simulink model "structuri_avansate_de_control"  (R2022b)
settings: Solver=FixedStepAuto  StartTime=0.0  StopTime=900  FixedStep=0.01  RelTol=1e-3
values from neighbouring files (symbols this model uses):
  C = 5.6    [CalculeProiect.m]
  h0 = 13.97    [CalculeProiect.m]
  h1 = 17.85    [CalculeProiect.m]
  k = 0.024    [CalculeProiect.m]
  k1 = 0.624    [CalculeProiect.m]
  k11 = k2*k2+4*(k-k3)*k1    (= 0.0616266)    [CalculeProiect.m]
  k12 = 8*(k-k3)    (= 0.1968)    [CalculeProiect.m]
  k13 = 2*(k-k3)    (= 0.0492)    [CalculeProiect.m]
  k2 = -0.015    [CalculeProiect.m]
  k3 = -0.0006    [CalculeProiect.m]
  kcompensare = (delta_h/(q1-q0))/(delta_h/delta_ua)    (= 0.185185185185)    [CalculeProiect.m]
  kp = (delta_h/3)/delta_ua    (= 2.58666666667)    [CalculeProiect.m]
  q0 = 20.97    [CalculeProiect.m]
undefined symbols (not defined in the file or in its folder): ki, ki1, ki2, kp1, kp2
libraries: slpidlib x6
(part 1 of 2)
settings Model: Creator=denis  LastModifiedBy=denis

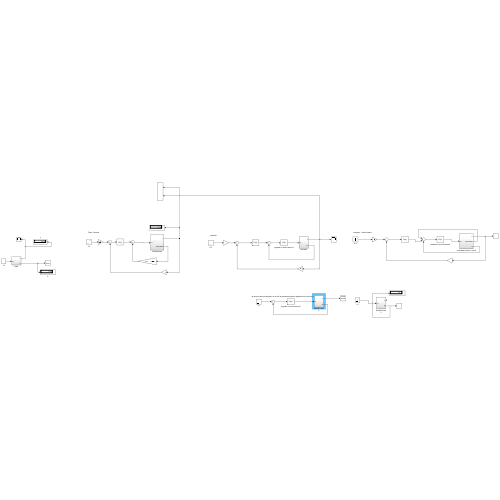
[thumbnail: Simulink's stored preview of the top-level diagram]
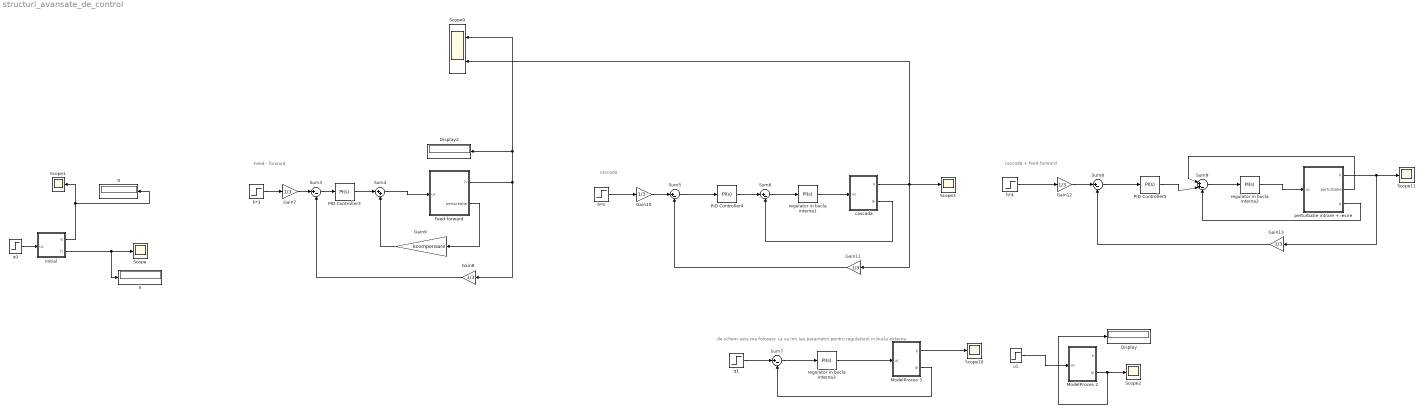
== system structuri_avansate_de_control ==
  note: de schem asta ma folosesc ca sa imi iau parametrii pentru regulatorul in bucla externa
  note: cascada
  note: Feed - forward
  note: cascada + feed-forward
  Display : Display
  Display2 : Display
  Feed-forward : Subsystem
  Gain{7..8,10..13} (6 alike) : Gain  Gain=1/3
  Gain9 : Gain  Gain=kcompensare
  ModelProces 2 : Subsystem
  ModelProces 3 : Subsystem
  PID Controller3 : slpidlib/PID Controller  Controller=PI  Form=Parallel  TimeDomain=Continuous-time  UseExternalTs=off  SampleTime=-1  IntegratorMethod=Forward Euler  FilterMethod=Forward Euler  ControllerParametersSource=internal  P=kp  I=ki  UseKiTs=off  D=0  N=100  UseFilter=on  TunerSelectOption=Transfer Function Based (PID Tuner App)  InitialConditionSource=internal  InitialConditionForIntegrator=4.4  InitialConditionForFilter=0  DifferentiatorICPrevScaledInput=0  ExternalReset=none  TrackingMode=off  Kt=1  LimitOutput=off  SatLimitsSource=internal  UpperSaturationLimit=inf  LowerSaturationLimit=-inf  LinearizeAsGain=on  AntiWindupMode=none  Kb=1  LimitIntegrator=off  UpperIntegratorSaturationLimit=inf  LowerIntegratorSaturationLimit=-inf  POutMin=[]  POutMax=[]  IOutMin=[]  IOutMax=[]  DOutMin=[]  DOutMax=[]  NOutMin=[]  NOutMax=[]  SumOutMin=[]  SumOutMax=[]  SaturationOutMin=[]  SaturationOutMax=[]  PParamMin=[]  PParamMax=[]  IParamMin=[]  IParamMax=[]  DParamMin=[]  DParamMax=[]  NParamMin=[]  NParamMax=[]  KbParamMin=[]  KbParamMax=[]  KtParamMin=[]  KtParamMax=[]  KbOutMin=[]  KbOutMax=[]  KtOutMin=[]  KtOutMax=[]  IntegratorOutMin=[]  IntegratorOutMax=[]  FilterOutMin=[]  FilterOutMax=[]  SumI1OutMin=[]  SumI1OutMax=[]  SumI2OutMin=[]  SumI2OutMax=[]  SumI3OutMin=[]  SumI3OutMax=[]  SumI4OutMin=[]  SumI4OutMax=[]  SumDOutMin=[]  SumDOutMax=[]  DifferentiatorOutMin=[]  DifferentiatorOutMax=[]  FilterDiffOutCoefMin=[]  FilterDiffOutCoefMax=[]  ReciprocalOutMin=[]  ReciprocalOutMax=[]  SumDenOutMin=[]  SumDenOutMax=[]  SumNumOutMin=[]  SumNumOutMax=[]  DivideOutMin=[]  DivideOutMax=[]  UdiffTsProdOutMin=[]  UdiffTsProdOutMax=[]  NTsProdOutMin=[]  NTsProdOutMax=[]  UintegralTsProdOutMin=[]  UintegralTsProdOutMax=[]  UngainTsProdOutMin=[]  UngainTsProdOutMax=[]  ClampingZeroOutDataTypeStr=Inherit: Inherit via back propagation  ClampingZeroOutMin=[]  ClampingZeroOutMax=[]  FilterDenConstantOutDataTypeStr=Inherit: Inherit via back propagation  FilterDenConstantOutMin=[]  FilterDenConstantOutMax=[]  PCopyOutDataTypeStr=Inherit: Inherit via back propagation  PCopyOutMin=[]  PCopyOutMax=[]  NCopyOutDataTypeStr=Inherit: Inherit via back propagation  NCopyOutMin=[]  NCopyOutMax=[]  IntegratorContinuousStateAttributes=''  IntegratorStateMustResolveToSignalObject=off  IntegratorRTWStateStorageClass=Auto  FilterContinuousStateAttributes=''  FilterStateMustResolveToSignalObject=off  FilterRTWStateStorageClass=Auto  ParallelPVariant=InternalParameters  IdealPVariant=Disabled  IVariant=InternalParameters  DVariant=Disabled  IntegratorVariant=Continuous  SatVariant=Disabled  AWVariant=Passthrough  PCopyVariant=Disabled  TRVariant=Disabled  FdbkBlocksVariant=Forward  IdealPFdbkVariant=Disabled  SatFdbkVariant=Disabled  DerivativeFilterVariant=Disabled  NVariant=Disabled  NCopyVariant=Disabled_SignalSpec  FilterICVariant=Disabled  IntegratorICVariant=InternalICs  ExternalResetVariant=Disabled  TRSumVariant=Passthrough  SumFdbkVariant=Disabled  SumVariant=Sum_PI  TsampFilterVariant=InternalTs  TsampNgainVariant=Passthrough  TsampIntegralVariant=Passthrough  ExternalSaturationOutDataTypeStr=Inherit: Same as second input
  PID Controller4 : slpidlib/PID Controller  Controller=PI  Form=Parallel  TimeDomain=Continuous-time  UseExternalTs=off  SampleTime=-1  IntegratorMethod=Forward Euler  FilterMethod=Forward Euler  ControllerParametersSource=internal  P=kp2  I=ki2  UseKiTs=off  D=0  N=100  UseFilter=on  TunerSelectOption=Transfer Function Based (PID Tuner App)  InitialConditionSource=internal  InitialConditionForIntegrator=20.97  InitialConditionForFilter=0  DifferentiatorICPrevScaledInput=0  ExternalReset=none  TrackingMode=off  Kt=1  LimitOutput=off  SatLimitsSource=internal  UpperSaturationLimit=inf  LowerSaturationLimit=-inf  LinearizeAsGain=on  AntiWindupMode=none  Kb=1  LimitIntegrator=off  UpperIntegratorSaturationLimit=inf  LowerIntegratorSaturationLimit=-inf  POutMin=[]  POutMax=[]  IOutMin=[]  IOutMax=[]  DOutMin=[]  DOutMax=[]  NOutMin=[]  NOutMax=[]  SumOutMin=[]  SumOutMax=[]  SaturationOutMin=[]  SaturationOutMax=[]  PParamMin=[]  PParamMax=[]  IParamMin=[]  IParamMax=[]  DParamMin=[]  DParamMax=[]  NParamMin=[]  NParamMax=[]  KbParamMin=[]  KbParamMax=[]  KtParamMin=[]  KtParamMax=[]  KbOutMin=[]  KbOutMax=[]  KtOutMin=[]  KtOutMax=[]  IntegratorOutMin=[]  IntegratorOutMax=[]  FilterOutMin=[]  FilterOutMax=[]  SumI1OutMin=[]  SumI1OutMax=[]  SumI2OutMin=[]  SumI2OutMax=[]  SumI3OutMin=[]  SumI3OutMax=[]  SumI4OutMin=[]  SumI4OutMax=[]  SumDOutMin=[]  SumDOutMax=[]  DifferentiatorOutMin=[]  DifferentiatorOutMax=[]  FilterDiffOutCoefMin=[]  FilterDiffOutCoefMax=[]  ReciprocalOutMin=[]  ReciprocalOutMax=[]  SumDenOutMin=[]  SumDenOutMax=[]  SumNumOutMin=[]  SumNumOutMax=[]  DivideOutMin=[]  DivideOutMax=[]  UdiffTsProdOutMin=[]  UdiffTsProdOutMax=[]  NTsProdOutMin=[]  NTsProdOutMax=[]  UintegralTsProdOutMin=[]  UintegralTsProdOutMax=[]  UngainTsProdOutMin=[]  UngainTsProdOutMax=[]  ClampingZeroOutDataTypeStr=Inherit: Inherit via back propagation  ClampingZeroOutMin=[]  ClampingZeroOutMax=[]  FilterDenConstantOutDataTypeStr=Inherit: Inherit via back propagation  FilterDenConstantOutMin=[]  FilterDenConstantOutMax=[]  PCopyOutDataTypeStr=Inherit: Inherit via back propagation  PCopyOutMin=[]  PCopyOutMax=[]  NCopyOutDataTypeStr=Inherit: Inherit via back propagation  NCopyOutMin=[]  NCopyOutMax=[]  IntegratorContinuousStateAttributes=''  IntegratorStateMustResolveToSignalObject=off  IntegratorRTWStateStorageClass=Auto  FilterContinuousStateAttributes=''  FilterStateMustResolveToSignalObject=off  FilterRTWStateStorageClass=Auto  ParallelPVariant=InternalParameters  IdealPVariant=Disabled  IVariant=InternalParameters  DVariant=Disabled  IntegratorVariant=Continuous  SatVariant=Disabled  AWVariant=Passthrough  PCopyVariant=Disabled  TRVariant=Disabled  FdbkBlocksVariant=Forward  IdealPFdbkVariant=Disabled  SatFdbkVariant=Disabled  DerivativeFilterVariant=Disabled  NVariant=Disabled  NCopyVariant=Disabled_SignalSpec  FilterICVariant=Disabled  IntegratorICVariant=InternalICs  ExternalResetVariant=Disabled  TRSumVariant=Passthrough  SumFdbkVariant=Disabled  SumVariant=Sum_PI  TsampFilterVariant=InternalTs  TsampNgainVariant=Passthrough  TsampIntegralVariant=Passthrough  ExternalSaturationOutDataTypeStr=Inherit: Same as second input
  PID Controller5 : slpidlib/PID Controller  Controller=PI  Form=Parallel  TimeDomain=Continuous-time  UseExternalTs=off  SampleTime=-1  IntegratorMethod=Forward Euler  FilterMethod=Forward Euler  ControllerParametersSource=internal  P=kp2  I=ki2  UseKiTs=off  D=0  N=100  UseFilter=on  TunerSelectOption=Transfer Function Based (PID Tuner App)  InitialConditionSource=internal  InitialConditionForIntegrator=q0  InitialConditionForFilter=0  DifferentiatorICPrevScaledInput=0  ExternalReset=none  TrackingMode=off  Kt=1  LimitOutput=off  SatLimitsSource=internal  UpperSaturationLimit=inf  LowerSaturationLimit=-inf  LinearizeAsGain=on  AntiWindupMode=none  Kb=1  LimitIntegrator=off  UpperIntegratorSaturationLimit=inf  LowerIntegratorSaturationLimit=-inf  POutMin=[]  POutMax=[]  IOutMin=[]  IOutMax=[]  DOutMin=[]  DOutMax=[]  NOutMin=[]  NOutMax=[]  SumOutMin=[]  SumOutMax=[]  SaturationOutMin=[]  SaturationOutMax=[]  PParamMin=[]  PParamMax=[]  IParamMin=[]  IParamMax=[]  DParamMin=[]  DParamMax=[]  NParamMin=[]  NParamMax=[]  KbParamMin=[]  KbParamMax=[]  KtParamMin=[]  KtParamMax=[]  KbOutMin=[]  KbOutMax=[]  KtOutMin=[]  KtOutMax=[]  IntegratorOutMin=[]  IntegratorOutMax=[]  FilterOutMin=[]  FilterOutMax=[]  SumI1OutMin=[]  SumI1OutMax=[]  SumI2OutMin=[]  SumI2OutMax=[]  SumI3OutMin=[]  SumI3OutMax=[]  SumI4OutMin=[]  SumI4OutMax=[]  SumDOutMin=[]  SumDOutMax=[]  DifferentiatorOutMin=[]  DifferentiatorOutMax=[]  FilterDiffOutCoefMin=[]  FilterDiffOutCoefMax=[]  ReciprocalOutMin=[]  ReciprocalOutMax=[]  SumDenOutMin=[]  SumDenOutMax=[]  SumNumOutMin=[]  SumNumOutMax=[]  DivideOutMin=[]  DivideOutMax=[]  UdiffTsProdOutMin=[]  UdiffTsProdOutMax=[]  NTsProdOutMin=[]  NTsProdOutMax=[]  UintegralTsProdOutMin=[]  UintegralTsProdOutMax=[]  UngainTsProdOutMin=[]  UngainTsProdOutMax=[]  ClampingZeroOutDataTypeStr=Inherit: Inherit via back propagation  ClampingZeroOutMin=[]  ClampingZeroOutMax=[]  FilterDenConstantOutDataTypeStr=Inherit: Inherit via back propagation  FilterDenConstantOutMin=[]  FilterDenConstantOutMax=[]  PCopyOutDataTypeStr=Inherit: Inherit via back propagation  PCopyOutMin=[]  PCopyOutMax=[]  NCopyOutDataTypeStr=Inherit: Inherit via back propagation  NCopyOutMin=[]  NCopyOutMax=[]  IntegratorContinuousStateAttributes=''  IntegratorStateMustResolveToSignalObject=off  IntegratorRTWStateStorageClass=Auto  FilterContinuousStateAttributes=''  FilterStateMustResolveToSignalObject=off  FilterRTWStateStorageClass=Auto  ParallelPVariant=InternalParameters  IdealPVariant=Disabled  IVariant=InternalParameters  DVariant=Disabled  IntegratorVariant=Continuous  SatVariant=Disabled  AWVariant=Passthrough  PCopyVariant=Disabled  TRVariant=Disabled  FdbkBlocksVariant=Forward  IdealPFdbkVariant=Disabled  SatFdbkVariant=Disabled  DerivativeFilterVariant=Disabled  NVariant=Disabled  NCopyVariant=Disabled_SignalSpec  FilterICVariant=Disabled  IntegratorICVariant=InternalICs  ExternalResetVariant=Disabled  TRSumVariant=Passthrough  SumFdbkVariant=Disabled  SumVariant=Sum_PI  TsampFilterVariant=InternalTs  TsampNgainVariant=Passthrough  TsampIntegralVariant=Passthrough  ExternalSaturationOutDataTypeStr=Inherit: Same as second input
  Scope{,1..3,10..11} (6 alike) : Scope
  Scope9 : Scope  NumInputPorts=2
  Sum{3,5..8} (5 alike) : Sum  Inputs=|+-
  Sum4 : Sum  Inputs=|++
  Sum9 : Sum  Inputs=|++-
  cascada : Subsystem
  h : Display
  h*3 : Step  Before=h0  After=h1  SampleTime=0
  h*4 : Step  Time=0  Before=h0  After=h1  SampleTime=0
  h*5 : Step  Time=0  Before=h0  After=h1  SampleTime=0
  initial : Subsystem
  perturbatie intrare + iesire : Subsystem
  q : Display
  q1 : Step  Time=0  Before=q0  After=29.02  SampleTime=0
  regulator in bucla interna1 : slpidlib/PID Controller  Controller=PI  Form=Parallel  TimeDomain=Continuous-time  UseExternalTs=off  SampleTime=-1  IntegratorMethod=Forward Euler  FilterMethod=Forward Euler  ControllerParametersSource=internal  P=kp1  I=ki1  UseKiTs=off  D=0  N=100  UseFilter=on  TunerSelectOption=Transfer Function Based (PID Tuner App)  InitialConditionSource=internal  InitialConditionForIntegrator=4.4  InitialConditionForFilter=0  DifferentiatorICPrevScaledInput=0  ExternalReset=none  TrackingMode=off  Kt=1  LimitOutput=off  SatLimitsSource=internal  UpperSaturationLimit=inf  LowerSaturationLimit=-inf  LinearizeAsGain=on  AntiWindupMode=none  Kb=1  LimitIntegrator=off  UpperIntegratorSaturationLimit=inf  LowerIntegratorSaturationLimit=-inf  POutMin=[]  POutMax=[]  IOutMin=[]  IOutMax=[]  DOutMin=[]  DOutMax=[]  NOutMin=[]  NOutMax=[]  SumOutMin=[]  SumOutMax=[]  SaturationOutMin=[]  SaturationOutMax=[]  PParamMin=[]  PParamMax=[]  IParamMin=[]  IParamMax=[]  DParamMin=[]  DParamMax=[]  NParamMin=[]  NParamMax=[]  KbParamMin=[]  KbParamMax=[]  KtParamMin=[]  KtParamMax=[]  KbOutMin=[]  KbOutMax=[]  KtOutMin=[]  KtOutMax=[]  IntegratorOutMin=[]  IntegratorOutMax=[]  FilterOutMin=[]  FilterOutMax=[]  SumI1OutMin=[]  SumI1OutMax=[]  SumI2OutMin=[]  SumI2OutMax=[]  SumI3OutMin=[]  SumI3OutMax=[]  SumI4OutMin=[]  SumI4OutMax=[]  SumDOutMin=[]  SumDOutMax=[]  DifferentiatorOutMin=[]  DifferentiatorOutMax=[]  FilterDiffOutCoefMin=[]  FilterDiffOutCoefMax=[]  ReciprocalOutMin=[]  ReciprocalOutMax=[]  SumDenOutMin=[]  SumDenOutMax=[]  SumNumOutMin=[]  SumNumOutMax=[]  DivideOutMin=[]  DivideOutMax=[]  UdiffTsProdOutMin=[]  UdiffTsProdOutMax=[]  NTsProdOutMin=[]  NTsProdOutMax=[]  UintegralTsProdOutMin=[]  UintegralTsProdOutMax=[]  UngainTsProdOutMin=[]  UngainTsProdOutMax=[]  ClampingZeroOutDataTypeStr=Inherit: Inherit via back propagation  ClampingZeroOutMin=[]  ClampingZeroOutMax=[]  FilterDenConstantOutDataTypeStr=Inherit: Inherit via back propagation  FilterDenConstantOutMin=[]  FilterDenConstantOutMax=[]  PCopyOutDataTypeStr=Inherit: Inherit via back propagation  PCopyOutMin=[]  PCopyOutMax=[]  NCopyOutDataTypeStr=Inherit: Inherit via back propagation  NCopyOutMin=[]  NCopyOutMax=[]  IntegratorContinuousStateAttributes=''  IntegratorStateMustResolveToSignalObject=off  IntegratorRTWStateStorageClass=Auto  FilterContinuousStateAttributes=''  FilterStateMustResolveToSignalObject=off  FilterRTWStateStorageClass=Auto  ParallelPVariant=InternalParameters  IdealPVariant=Disabled  IVariant=InternalParameters  DVariant=Disabled  IntegratorVariant=Continuous  SatVariant=Disabled  AWVariant=Passthrough  PCopyVariant=Disabled  TRVariant=Disabled  FdbkBlocksVariant=Forward  IdealPFdbkVariant=Disabled  SatFdbkVariant=Disabled  DerivativeFilterVariant=Disabled  NVariant=Disabled  NCopyVariant=Disabled_SignalSpec  FilterICVariant=Disabled  IntegratorICVariant=InternalICs  ExternalResetVariant=Disabled  TRSumVariant=Passthrough  SumFdbkVariant=Disabled  SumVariant=Sum_PI  TsampFilterVariant=InternalTs  TsampNgainVariant=Passthrough  TsampIntegralVariant=Passthrough  ExternalSaturationOutDataTypeStr=Inherit: Same as second input
  regulator in bucla interna2 : slpidlib/PID Controller  Controller=PI  Form=Parallel  TimeDomain=Continuous-time  UseExternalTs=off  SampleTime=-1  IntegratorMethod=Forward Euler  FilterMethod=Forward Euler  ControllerParametersSource=internal  P=kp1  I=ki1  UseKiTs=off  D=0  N=100  UseFilter=on  TunerSelectOption=Transfer Function Based (PID Tuner App)  InitialConditionSource=internal  InitialConditionForIntegrator=4.4  InitialConditionForFilter=0  DifferentiatorICPrevScaledInput=0  ExternalReset=none  TrackingMode=off  Kt=1  LimitOutput=off  SatLimitsSource=internal  UpperSaturationLimit=inf  LowerSaturationLimit=-inf  LinearizeAsGain=on  AntiWindupMode=none  Kb=1  LimitIntegrator=off  UpperIntegratorSaturationLimit=inf  LowerIntegratorSaturationLimit=-inf  POutMin=[]  POutMax=[]  IOutMin=[]  IOutMax=[]  DOutMin=[]  DOutMax=[]  NOutMin=[]  NOutMax=[]  SumOutMin=[]  SumOutMax=[]  SaturationOutMin=[]  SaturationOutMax=[]  PParamMin=[]  PParamMax=[]  IParamMin=[]  IParamMax=[]  DParamMin=[]  DParamMax=[]  NParamMin=[]  NParamMax=[]  KbParamMin=[]  KbParamMax=[]  KtParamMin=[]  KtParamMax=[]  KbOutMin=[]  KbOutMax=[]  KtOutMin=[]  KtOutMax=[]  IntegratorOutMin=[]  IntegratorOutMax=[]  FilterOutMin=[]  FilterOutMax=[]  SumI1OutMin=[]  SumI1OutMax=[]  SumI2OutMin=[]  SumI2OutMax=[]  SumI3OutMin=[]  SumI3OutMax=[]  SumI4OutMin=[]  SumI4OutMax=[]  SumDOutMin=[]  SumDOutMax=[]  DifferentiatorOutMin=[]  DifferentiatorOutMax=[]  FilterDiffOutCoefMin=[]  FilterDiffOutCoefMax=[]  ReciprocalOutMin=[]  ReciprocalOutMax=[]  SumDenOutMin=[]  SumDenOutMax=[]  SumNumOutMin=[]  SumNumOutMax=[]  DivideOutMin=[]  DivideOutMax=[]  UdiffTsProdOutMin=[]  UdiffTsProdOutMax=[]  NTsProdOutMin=[]  NTsProdOutMax=[]  UintegralTsProdOutMin=[]  UintegralTsProdOutMax=[]  UngainTsProdOutMin=[]  UngainTsProdOutMax=[]  ClampingZeroOutDataTypeStr=Inherit: Inherit via back propagation  ClampingZeroOutMin=[]  ClampingZeroOutMax=[]  FilterDenConstantOutDataTypeStr=Inherit: Inherit via back propagation  FilterDenConstantOutMin=[]  FilterDenConstantOutMax=[]  PCopyOutDataTypeStr=Inherit: Inherit via back propagation  PCopyOutMin=[]  PCopyOutMax=[]  NCopyOutDataTypeStr=Inherit: Inherit via back propagation  NCopyOutMin=[]  NCopyOutMax=[]  IntegratorContinuousStateAttributes=''  IntegratorStateMustResolveToSignalObject=off  IntegratorRTWStateStorageClass=Auto  FilterContinuousStateAttributes=''  FilterStateMustResolveToSignalObject=off  FilterRTWStateStorageClass=Auto  ParallelPVariant=InternalParameters  IdealPVariant=Disabled  IVariant=InternalParameters  DVariant=Disabled  IntegratorVariant=Continuous  SatVariant=Disabled  AWVariant=Passthrough  PCopyVariant=Disabled  TRVariant=Disabled  FdbkBlocksVariant=Forward  IdealPFdbkVariant=Disabled  SatFdbkVariant=Disabled  DerivativeFilterVariant=Disabled  NVariant=Disabled  NCopyVariant=Disabled_SignalSpec  FilterICVariant=Disabled  IntegratorICVariant=InternalICs  ExternalResetVariant=Disabled  TRSumVariant=Passthrough  SumFdbkVariant=Disabled  SumVariant=Sum_PI  TsampFilterVariant=InternalTs  TsampNgainVariant=Passthrough  TsampIntegralVariant=Passthrough  ExternalSaturationOutDataTypeStr=Inherit: Same as second input
  regulator in bucla interna3 : slpidlib/PID Controller  Controller=PI  Form=Parallel  TimeDomain=Continuous-time  UseExternalTs=off  SampleTime=-1  IntegratorMethod=Forward Euler  FilterMethod=Forward Euler  ControllerParametersSource=internal  P=kp1  I=ki1  UseKiTs=off  D=0  N=100  UseFilter=on  TunerSelectOption=Transfer Function Based (PID Tuner App)  InitialConditionSource=internal  InitialConditionForIntegrator=4.4  InitialConditionForFilter=0  DifferentiatorICPrevScaledInput=0  ExternalReset=none  TrackingMode=off  Kt=1  LimitOutput=off  SatLimitsSource=internal  UpperSaturationLimit=inf  LowerSaturationLimit=-inf  LinearizeAsGain=on  AntiWindupMode=none  Kb=1  LimitIntegrator=off  UpperIntegratorSaturationLimit=inf  LowerIntegratorSaturationLimit=-inf  POutMin=[]  POutMax=[]  IOutMin=[]  IOutMax=[]  DOutMin=[]  DOutMax=[]  NOutMin=[]  NOutMax=[]  SumOutMin=[]  SumOutMax=[]  SaturationOutMin=[]  SaturationOutMax=[]  PParamMin=[]  PParamMax=[]  IParamMin=[]  IParamMax=[]  DParamMin=[]  DParamMax=[]  NParamMin=[]  NParamMax=[]  KbParamMin=[]  KbParamMax=[]  KtParamMin=[]  KtParamMax=[]  KbOutMin=[]  KbOutMax=[]  KtOutMin=[]  KtOutMax=[]  IntegratorOutMin=[]  IntegratorOutMax=[]  FilterOutMin=[]  FilterOutMax=[]  SumI1OutMin=[]  SumI1OutMax=[]  SumI2OutMin=[]  SumI2OutMax=[]  SumI3OutMin=[]  SumI3OutMax=[]  SumI4OutMin=[]  SumI4OutMax=[]  SumDOutMin=[]  SumDOutMax=[]  DifferentiatorOutMin=[]  DifferentiatorOutMax=[]  FilterDiffOutCoefMin=[]  FilterDiffOutCoefMax=[]  ReciprocalOutMin=[]  ReciprocalOutMax=[]  SumDenOutMin=[]  SumDenOutMax=[]  SumNumOutMin=[]  SumNumOutMax=[]  DivideOutMin=[]  DivideOutMax=[]  UdiffTsProdOutMin=[]  UdiffTsProdOutMax=[]  NTsProdOutMin=[]  NTsProdOutMax=[]  UintegralTsProdOutMin=[]  UintegralTsProdOutMax=[]  UngainTsProdOutMin=[]  UngainTsProdOutMax=[]  ClampingZeroOutDataTypeStr=Inherit: Inherit via back propagation  ClampingZeroOutMin=[]  ClampingZeroOutMax=[]  FilterDenConstantOutDataTypeStr=Inherit: Inherit via back propagation  FilterDenConstantOutMin=[]  FilterDenConstantOutMax=[]  PCopyOutDataTypeStr=Inherit: Inherit via back propagation  PCopyOutMin=[]  PCopyOutMax=[]  NCopyOutDataTypeStr=Inherit: Inherit via back propagation  NCopyOutMin=[]  NCopyOutMax=[]  IntegratorContinuousStateAttributes=''  IntegratorStateMustResolveToSignalObject=off  IntegratorRTWStateStorageClass=Auto  FilterContinuousStateAttributes=''  FilterStateMustResolveToSignalObject=off  FilterRTWStateStorageClass=Auto  ParallelPVariant=InternalParameters  IdealPVariant=Disabled  IVariant=InternalParameters  DVariant=Disabled  IntegratorVariant=Continuous  SatVariant=Disabled  AWVariant=Passthrough  PCopyVariant=Disabled  TRVariant=Disabled  FdbkBlocksVariant=Forward  IdealPFdbkVariant=Disabled  SatFdbkVariant=Disabled  DerivativeFilterVariant=Disabled  NVariant=Disabled  NCopyVariant=Disabled_SignalSpec  FilterICVariant=Disabled  IntegratorICVariant=InternalICs  ExternalResetVariant=Disabled  TRSumVariant=Passthrough  SumFdbkVariant=Disabled  SumVariant=Sum_PI  TsampFilterVariant=InternalTs  TsampNgainVariant=Passthrough  TsampIntegralVariant=Passthrough  ExternalSaturationOutDataTypeStr=Inherit: Same as second input
  u0 : Step  Time=0  Before=4.4  After=4.9  SampleTime=0
  u1 : Step  Time=0  Before=4.4  After=4.9  SampleTime=0
  wires:
  Sum4/1 -> Feed-forward/1(uc)
  ModelProces 3/2(qi) -> Sum7/2
  cascada/1(h) -> Scope9/2, Scope3/1, Gain11/1
  ModelProces 2/2(qi) -> Display/1, Scope2/1
  Sum3/1 -> PID Controller3/1
  Gain12/1 -> Sum8/1
  Sum9/1 -> regulator in bucla interna2/1
  Gain11/1 -> Sum5/2
  regulator in bucla interna3/1 -> ModelProces 3/1(uc)
  initial/2(h) -> Scope/1, h/1
  Feed-forward/2(perturbatie) -> Gain9/1
  PID Controller3/1 -> Sum4/1
  Gain10/1 -> Sum5/1
  initial/1(q) -> Scope1/1, q/1
  h*3/1 -> Gain7/1
  Gain7/1 -> Sum3/1
  Sum6/1 -> regulator in bucla interna1/1
  regulator in bucla interna1/1 -> cascada/1(uc)
  ModelProces 3/1(h) -> Scope10/1
  perturbatie intrare + iesire/1(h) -> Gain13/1, Scope11/1
  h*5/1 -> Gain10/1
  Sum5/1 -> PID Controller4/1
  q1/1 -> Sum7/1
  Gain13/1 -> Sum8/2
  Gain8/1 -> Sum3/2
  PID Controller4/1 -> Sum6/1
  Sum7/1 -> regulator in bucla interna3/1
  perturbatie intrare + iesire/3(q) -> Sum9/3
  u1/1 -> ModelProces 2/1(uc)
  perturbatie intrare + iesire/2(perturbatie) -> Sum9/1
  u0/1 -> initial/1(uc)
  Gain9/1 -> Sum4/2
  Sum8/1 -> PID Controller5/1
  cascada/2(qi) -> Sum6/2
  Feed-forward/1(h) -> Gain8/1, Scope9/1, Display2/1
  regulator in bucla interna2/1 -> perturbatie intrare + iesire/1(uc)
  PID Controller5/1 -> Sum9/2
  h*4/1 -> Gain12/1

== system structuri_avansate_de_control/Feed-forward ==
  uc : Inport
  Amplificator : Subsystem
  Curent rotoric : Subsystem
  Filtru : Subsystem
  Motor : Subsystem
  Pompa : Subsystem
  Randament pompa : Subsystem
  Rezervor : Subsystem
  h : Outport
  perturbatie : Outport  Port=2
  wires:
  Filtru/1(q2) -> Curent rotoric/2(q), Randament pompa/1(q), Rezervor/1(q)
  Rezervor/1(h) -> h/1, Curent rotoric/1(h), Pompa/2(h)
  Motor/1(kn) -> Pompa/1(kn)
  Curent rotoric/1(im) -> Motor/2(im)
  Amplificator/1(um) -> Motor/1(um), Curent rotoric/4(um), Randament pompa/2(um)
  uc/1 -> Amplificator/1(ua)
  Randament pompa/1(eta) -> Curent rotoric/3(eta)
  Pompa/1(q) -> Filtru/1(q1)
  Rezervor/2(perturbatie) -> perturbatie/1

== system structuri_avansate_de_control/ModelProces 2 ==
  uc : Inport
  "Amplificator " : Subsystem
  Curentul_rotoric : Subsystem
  Filtru : Subsystem
  "Motor " : Subsystem
  Pompa : Subsystem
  Randament : Subsystem
  Rezervor : Subsystem
  perturbatie k : Step  Time=300  After=0.03  SampleTime=0
  h : Outport
  qi : Outport  Port=2
  wires:
  "Amplificator "/1("um ") -> "Motor "/1(um), Randament/2(um), Curentul_rotoric/4(um)
  Filtru/1(q_f) -> Rezervor/1(q), qi/1, Randament/1("q "), Curentul_rotoric/1(q)
  Rezervor/1(h) -> h/1, Curentul_rotoric/3(h), Pompa/1(h)
  Curentul_rotoric/1(im) -> "Motor "/2(im)
  Randament/1("eta ") -> Curentul_rotoric/2(eta)
  uc/1 -> "Amplificator "/1(ua)
  Pompa/1(q) -> Filtru/1(q)
  perturbatie k/1 -> Pompa/2(perturbatie k)
  "Motor "/1(kn) -> Pompa/3(kn)

== system structuri_avansate_de_control/ModelProces 3 ==
  uc : Inport
  "Amplificator " : Subsystem
  Curentul_rotoric : Subsystem
  Filtru : Subsystem
  "Motor " : Subsystem
  Pompa : Subsystem
  Randament : Subsystem
  Rezervor : Subsystem
  perturbatie k : Step  Time=300  After=0.03  SampleTime=0
  h : Outport
  qi : Outport  Port=2
  wires:
  "Amplificator "/1("um ") -> "Motor "/1(um), Randament/2(um), Curentul_rotoric/4(um)
  Filtru/1(q_f) -> Rezervor/1(q), qi/1, Randament/1("q "), Curentul_rotoric/1(q)
  Rezervor/1(h) -> h/1, Curentul_rotoric/3(h), Pompa/1(h)
  Curentul_rotoric/1(im) -> "Motor "/2(im)
  Randament/1("eta ") -> Curentul_rotoric/2(eta)
  uc/1 -> "Amplificator "/1(ua)
  Pompa/1(q) -> Filtru/1(q)
  perturbatie k/1 -> Pompa/2(perturbatie k)
  "Motor "/1(kn) -> Pompa/3(kn)

== system structuri_avansate_de_control/cascada ==
  uc : Inport
  "Amplificator " : Subsystem
  Curentul_rotoric : Subsystem
  Filtru : Subsystem
  "Motor " : Subsystem
  Pompa : Subsystem
  Randament : Subsystem
  Rezervor : Subsystem
  perturbatie k : Step  Time=300  After=-0.02  SampleTime=0
  h : Outport
  qi : Outport  Port=2
  wires:
  "Amplificator "/1("um ") -> "Motor "/1(um), Randament/2(um), Curentul_rotoric/4(um)
  Filtru/1(q_f) -> Rezervor/1(q), qi/1, Randament/1("q "), Curentul_rotoric/1(q)
  Rezervor/1(h) -> h/1, Curentul_rotoric/3(h), Pompa/1(h)
  Curentul_rotoric/1(im) -> "Motor "/2(im)
  Randament/1("eta ") -> Curentul_rotoric/2(eta)
  uc/1 -> "Amplificator "/1(ua)
  Pompa/1(q) -> Filtru/1(q)
  perturbatie k/1 -> Pompa/2(perturbatie k)
  "Motor "/1(kn) -> Pompa/3(kn)

== system structuri_avansate_de_control/initial ==
  uc : Inport
  Amplificator : Subsystem
  Curent rotoric : Subsystem
  Filtru : Subsystem
  Motor : Subsystem
  Pompa : Subsystem
  Randament pompa : Subsystem
  Rezervor : Subsystem
  q : Outport
  h : Outport  Port=2
  wires:
  Filtru/1(q2) -> Curent rotoric/2(q), Randament pompa/1(q), Rezervor/1(ln1), q/1
  Rezervor/1(h) -> h/1, Curent rotoric/1(h), Pompa/2(h)
  Motor/1(kn) -> Pompa/1(kn)
  Curent rotoric/1(im) -> Motor/2(im)
  Amplificator/1(um) -> Motor/1(um), Curent rotoric/4(um), Randament pompa/2(um)
  uc/1 -> Amplificator/1(ua)
  Randament pompa/1(eta) -> Curent rotoric/3(eta)
  Pompa/1(q) -> Filtru/1(q1)

== system structuri_avansate_de_control/perturbatie intrare + iesire ==
  uc : Inport
  Amplificator : Subsystem
  Curent rotoric : Subsystem
  Filtru : Subsystem
  Motor : Subsystem
  Pompa : Subsystem
  Randament pompa : Subsystem
  Rezervor : Subsystem
  Step : Step  Time=300  After=-0.01  SampleTime=0
  h : Outport
  perturbatie : Outport  Port=2
  q : Outport  Port=3
  wires:
  Filtru/1(q2) -> Curent rotoric/2(q), Randament pompa/1(q), Rezervor/1(q), q/1
  Rezervor/1(h) -> h/1, Pompa/3(h), Curent rotoric/1(h)
  Curent rotoric/1(im) -> Motor/2(im)
  Amplificator/1(um) -> Motor/1(um), Curent rotoric/4(um), Randament pompa/2(um)
  uc/1 -> Amplificator/1(ua)
  Randament pompa/1(eta) -> Curent rotoric/3(eta)
  Pompa/1(q) -> Filtru/1(q1)
  Rezervor/2(perturbatie) -> perturbatie/1
  Motor/1(kn) -> Pompa/1(kn)
  Step/1 -> Pompa/2(perturbatie k)

== system structuri_avansate_de_control/Feed-forward/Amplificator ==
  ua : Inport
  Constant : Constant  Value=8.1
  Gain : Gain  Gain=2.2
  Gain1 : Gain  Gain=5
  Gain2 : Gain  Gain=2.2
  Saturation : Saturate  UpperLimit=22  LowerLimit=0
  Sum : Sum  Inputs=|++
  Sum1 : Sum  Inputs=|+-
  Switch : Switch  Criteria=u2 > Threshold  Threshold=8.1  SaturateOnIntegerOverflow=off  InputSameDT=off
  um : Outport
  wires:
  Gain/1 -> Switch/3
  Sum1/1 -> Gain1/1
  ua/1 -> Gain/1, Sum1/1, Gain2/1, Switch/2
  Switch/1 -> Saturation/1
  Gain1/1 -> Sum/2
  Saturation/1 -> um/1
  Constant/1 -> Sum1/2
  Gain2/1 -> Sum/1
  Sum/1 -> Switch/1

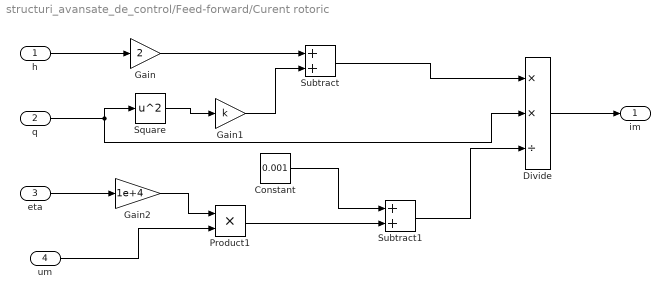
== system structuri_avansate_de_control/Feed-forward/Curent rotoric ==
  h : Inport
  q : Inport  Port=2
  eta : Inport  Port=3
  um : Inport  Port=4
  Constant : Constant  Value=0.001
  Divide : Product  Inputs=**/
  Gain : Gain  Gain=2
  Gain1 : Gain  Gain=k
  Gain2 : Gain  Gain=1e+4
  Product1 : Product
  Square : Math  Operator=square
  Subtract : Sum
  Subtract1 : Sum
  im : Outport
  wires:
  h/1 -> Gain/1
  Divide/1 -> im/1
  q/1 -> Divide/2, Square/1
  eta/1 -> Gain2/1
  um/1 -> Product1/2
  Gain2/1 -> Product1/1
  Subtract/1 -> Divide/1
  Constant/1 -> Subtract1/1
  Product1/1 -> Subtract1/2
  Subtract1/1 -> Divide/3
  Gain/1 -> Subtract/1
  Gain1/1 -> Subtract/2
  Square/1 -> Gain1/1

== system structuri_avansate_de_control/Feed-forward/Filtru ==
  q1 : Inport
  Integrator1 : Integrator  InitialCondition=q0
  Sum1 : Sum  Inputs=|+-
  q2 : Outport
  wires:
  Integrator1/1 -> q2/1, Sum1/2
  q1/1 -> Sum1/1
  Sum1/1 -> Integrator1/1

== system structuri_avansate_de_control/Feed-forward/Motor ==
  um : Inport
  im : Inport  Port=2
  Add : Sum  Inputs=+-
  Rm : Gain  Gain=3
  kn : Outport
  wires:
  Rm/1 -> Add/2
  um/1 -> Add/1
  im/1 -> Rm/1
  Add/1 -> kn/1

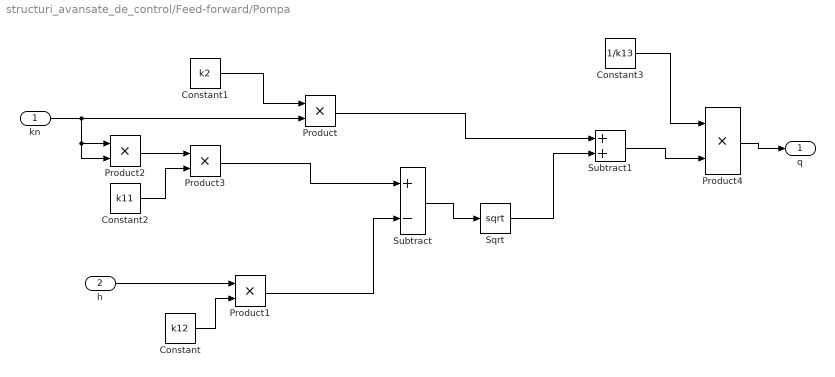
== system structuri_avansate_de_control/Feed-forward/Pompa ==
  kn : Inport
  h : Inport  Port=2
  Constant : Constant  Value=k12
  Constant1 : Constant  Value=k2
  Constant2 : Constant  Value=k11
  Constant3 : Constant  Value=1/k13
  Product{,1..4} (5 alike) : Product
  Sqrt : Sqrt
  Subtract : Sum  Inputs=+-
  Subtract1 : Sum
  q : Outport
  wires:
  Subtract/1 -> Sqrt/1
  Sqrt/1 -> Subtract1/2
  h/1 -> Product1/1
  Product1/1 -> Subtract/2
  Constant/1 -> Product1/2
  Constant1/1 -> Product/1
  kn/1 -> Product2/2, Product2/1, Product/2
  Product/1 -> Subtract1/1
  Product2/1 -> Product3/1
  Constant2/1 -> Product3/2
  Product3/1 -> Subtract/1
  Constant3/1 -> Product4/1
  Subtract1/1 -> Product4/2
  Product4/1 -> q/1

== system structuri_avansate_de_control/Feed-forward/Randament pompa ==
  q : Inport
  um : Inport  Port=2
  Gain : Gain  Gain=8e-5
  Product : Product
  eta : Outport
  wires:
  um/1 -> Gain/1
  Gain/1 -> Product/2
  q/1 -> Product/1
  Product/1 -> eta/1

== system structuri_avansate_de_control/Feed-forward/Rezervor ==
  q : Inport
  Add : Sum
  Constant : Constant  Value=C
  Gain : Gain  Gain=1/332.5
  Integrator1 : Integrator  InitialCondition=h0
  Product : Product
  Product1 : Product
  Scope : Scope
  Sqrt : Sqrt
  Step : Step  Time=500  After=0.11  SampleTime=0
  Sum1 : Sum  Inputs=|+-
  h : Outport
  perturbatie : Outport  Port=2
  wires:
  Gain/1 -> Integrator1/1
  Integrator1/1 -> Sqrt/1, h/1
  Sum1/1 -> Gain/1
  q/1 -> Sum1/1
  Sqrt/1 -> Product1/1, Product/1
  Product/1 -> Sum1/2, Scope/1
  Product1/1 -> perturbatie/1
  Constant/1 -> Add/2
  Step/1 -> Product1/2, Add/1
  Add/1 -> Product/2

== system structuri_avansate_de_control/ModelProces 2/Amplificator  ==
  ua : Inport
  Constant : Constant  Value=8.1
  Gain : Gain  Gain=2.2
  Gain1 : Gain  Gain=2.2
  Gain2 : Gain  Gain=5
  Saturation : Saturate  UpperLimit=22  LowerLimit=0
  Sum : Sum  Inputs=|++
  Sum1 : Sum  Inputs=|+-
  Switch : Switch  Threshold=8.1  SaturateOnIntegerOverflow=off  InputSameDT=off
  "um " : Outport
  wires:
  Sum1/1 -> Gain2/1
  ua/1 -> Switch/2, Gain/1, Sum1/1, Gain1/1
  Gain2/1 -> Sum/2
  Gain1/1 -> Sum/1
  Sum/1 -> Switch/1
  Gain/1 -> Switch/3
  Constant/1 -> Sum1/2
  Switch/1 -> Saturation/1
  Saturation/1 -> "um "/1

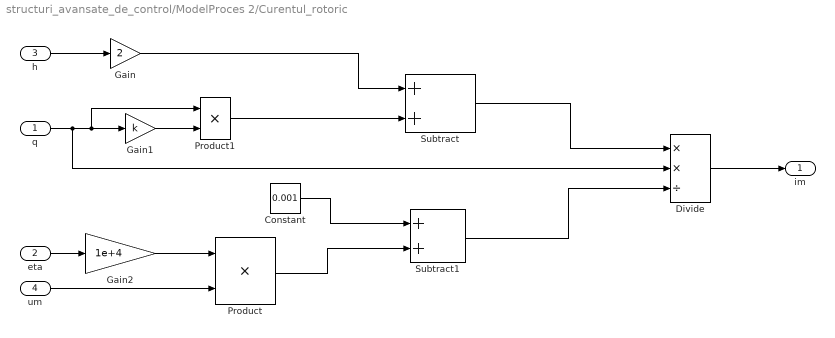
== system structuri_avansate_de_control/ModelProces 2/Curentul_rotoric ==
  q : Inport
  eta : Inport  Port=2
  h : Inport  Port=3
  um : Inport  Port=4
  Constant : Constant  Value=0.001
  Divide : Product  Inputs=**/
  Gain : Gain  Gain=2
  Gain1 : Gain  Gain=k
  Gain2 : Gain  Gain=1e+4
  Product : Product
  Product1 : Product
  Subtract : Sum
  Subtract1 : Sum
  im : Outport
  wires:
  h/1 -> Gain/1
  Gain/1 -> Subtract/1
  q/1 -> Divide/2, Product1/1, Gain1/1
  Gain1/1 -> Product1/2
  Product1/1 -> Subtract/2
  eta/1 -> Gain2/1
  Gain2/1 -> Product/1
  um/1 -> Product/2
  Constant/1 -> Subtract1/1
  Product/1 -> Subtract1/2
  Divide/1 -> im/1
  Subtract/1 -> Divide/1
  Subtract1/1 -> Divide/3

== system structuri_avansate_de_control/ModelProces 2/Filtru ==
  q : Inport
  Integrator : Integrator  InitialCondition=20.97
  Sum : Sum  Inputs=|+-
  q_f : Outport
  wires:
  Integrator/1 -> Sum/2, q_f/1
  q/1 -> Sum/1
  Sum/1 -> Integrator/1

== system structuri_avansate_de_control/ModelProces 2/Motor  ==
  um : Inport
  im : Inport  Port=2
  Add : Sum  Inputs=+-
  Rm : Gain  Gain=3
  kn : Outport
  wires:
  Rm/1 -> Add/2
  um/1 -> Add/1
  im/1 -> Rm/1
  Add/1 -> kn/1

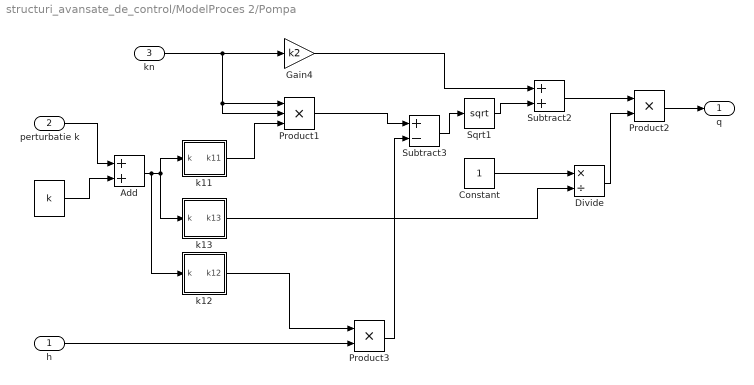
== system structuri_avansate_de_control/ModelProces 2/Pompa ==
  h : Inport
  perturbatie k : Inport  Port=2
  kn : Inport  Port=3
  " " : Constant  Value=k
  Add : Sum
  Constant : Constant
  Divide : Product  Inputs=*/
  Gain4 : Gain  Gain=k2
  Product1 : Product  Inputs=3
  Product2 : Product
  Product3 : Product
  Sqrt1 : Sqrt
  Subtract2 : Sum
  Subtract3 : Sum  Inputs=+-
  "k11 " : Subsystem
  k12 : Subsystem
  k13 : Subsystem
  q : Outport
  wires:
  Product2/1 -> q/1
  Divide/1 -> Product2/2
  Sqrt1/1 -> Subtract2/2
  k13/1(k13) -> Divide/2
  Constant/1 -> Divide/1
  "k11 "/1(k11) -> Product1/3
  Product3/1 -> Subtract3/2
  k12/1(k12) -> Product3/1
  Subtract2/1 -> Product2/1
  Add/1 -> k12/1(k), k13/1(k), "k11 "/1(k)
  perturbatie k/1 -> Add/1
  " "/1 -> Add/2
  Subtract3/1 -> Sqrt1/1
  kn/1 -> Product1/2, Product1/1, Gain4/1
  h/1 -> Product3/2
  Gain4/1 -> Subtract2/1
  Product1/1 -> Subtract3/1

== system structuri_avansate_de_control/ModelProces 2/Randament ==
  "q " : Inport
  um : Inport  Port=2
  Gain : Gain  Gain=8e-5
  Product : Product
  "eta " : Outport
  wires:
  um/1 -> Gain/1
  Gain/1 -> Product/2
  "q "/1 -> Product/1
  Product/1 -> "eta "/1

== system structuri_avansate_de_control/ModelProces 2/Rezervor ==
  q : Inport
  Gain : Gain  Gain=1/332.5
  Integrator : Integrator  InitialCondition=13.98
  Product : Product
  Sqrt : Sqrt
  Sum : Sum  Inputs=|+-
  c : Constant  Value=C
  h : Outport
  wires:
  Sum/1 -> Gain/1
  Sqrt/1 -> Product/1
  q/1 -> Sum/1
  Gain/1 -> Integrator/1
  Product/1 -> Sum/2
  c/1 -> Product/2
  Integrator/1 -> h/1, Sqrt/1

== system structuri_avansate_de_control/ModelProces 3/Amplificator  ==
  ua : Inport
  Constant : Constant  Value=8.1
  Gain : Gain  Gain=2.2
  Gain1 : Gain  Gain=2.2
  Gain2 : Gain  Gain=5
  Saturation : Saturate  UpperLimit=22  LowerLimit=0
  Sum : Sum  Inputs=|++
  Sum1 : Sum  Inputs=|+-
  Switch : Switch  Threshold=8.1  SaturateOnIntegerOverflow=off  InputSameDT=off
  "um " : Outport
  wires:
  Sum1/1 -> Gain2/1
  ua/1 -> Switch/2, Gain/1, Sum1/1, Gain1/1
  Gain2/1 -> Sum/2
  Gain1/1 -> Sum/1
  Sum/1 -> Switch/1
  Gain/1 -> Switch/3
  Constant/1 -> Sum1/2
  Switch/1 -> Saturation/1
  Saturation/1 -> "um "/1

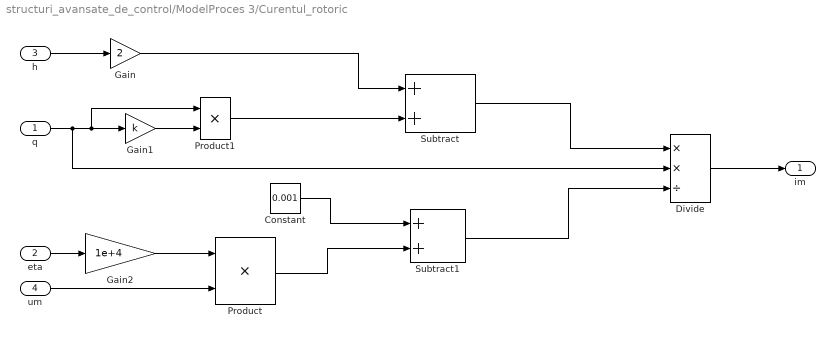
== system structuri_avansate_de_control/ModelProces 3/Curentul_rotoric ==
  q : Inport
  eta : Inport  Port=2
  h : Inport  Port=3
  um : Inport  Port=4
  Constant : Constant  Value=0.001
  Divide : Product  Inputs=**/
  Gain : Gain  Gain=2
  Gain1 : Gain  Gain=k
  Gain2 : Gain  Gain=1e+4
  Product : Product
  Product1 : Product
  Subtract : Sum
  Subtract1 : Sum
  im : Outport
  wires:
  h/1 -> Gain/1
  Gain/1 -> Subtract/1
  q/1 -> Divide/2, Product1/1, Gain1/1
  Gain1/1 -> Product1/2
  Product1/1 -> Subtract/2
  eta/1 -> Gain2/1
  Gain2/1 -> Product/1
  um/1 -> Product/2
  Constant/1 -> Subtract1/1
  Product/1 -> Subtract1/2
  Divide/1 -> im/1
  Subtract/1 -> Divide/1
  Subtract1/1 -> Divide/3

== system structuri_avansate_de_control/ModelProces 3/Filtru ==
  q : Inport
  Integrator : Integrator  InitialCondition=20.97
  Sum : Sum  Inputs=|+-
  q_f : Outport
  wires:
  Integrator/1 -> Sum/2, q_f/1
  q/1 -> Sum/1
  Sum/1 -> Integrator/1

== system structuri_avansate_de_control/ModelProces 3/Motor  ==
  um : Inport
  im : Inport  Port=2
  Add : Sum  Inputs=+-
  Rm : Gain  Gain=3
  kn : Outport
  wires:
  Rm/1 -> Add/2
  um/1 -> Add/1
  im/1 -> Rm/1
  Add/1 -> kn/1

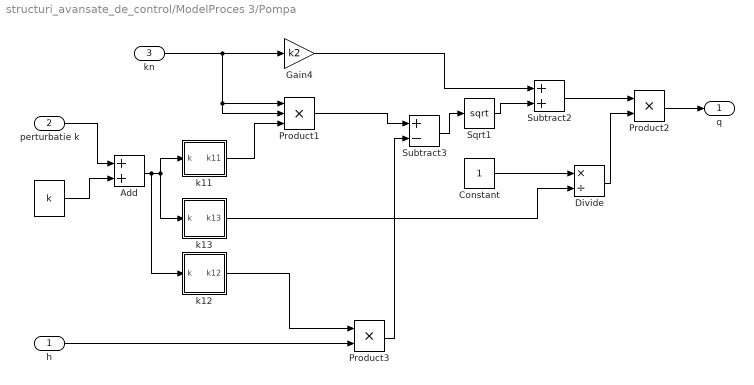
== system structuri_avansate_de_control/ModelProces 3/Pompa ==
  h : Inport
  perturbatie k : Inport  Port=2
  kn : Inport  Port=3
  " " : Constant  Value=k
  Add : Sum
  Constant : Constant
  Divide : Product  Inputs=*/
  Gain4 : Gain  Gain=k2
  Product1 : Product  Inputs=3
  Product2 : Product
  Product3 : Product
  Sqrt1 : Sqrt
  Subtract2 : Sum
  Subtract3 : Sum  Inputs=+-
  "k11 " : Subsystem
  k12 : Subsystem
  k13 : Subsystem
  q : Outport
  wires:
  Product2/1 -> q/1
  Divide/1 -> Product2/2
  Sqrt1/1 -> Subtract2/2
  k13/1(k13) -> Divide/2
  Constant/1 -> Divide/1
  "k11 "/1(k11) -> Product1/3
  Product3/1 -> Subtract3/2
  k12/1(k12) -> Product3/1
  Subtract2/1 -> Product2/1
  Add/1 -> k12/1(k), k13/1(k), "k11 "/1(k)
  perturbatie k/1 -> Add/1
  " "/1 -> Add/2
  Subtract3/1 -> Sqrt1/1
  kn/1 -> Product1/2, Product1/1, Gain4/1
  h/1 -> Product3/2
  Gain4/1 -> Subtract2/1
  Product1/1 -> Subtract3/1

== system structuri_avansate_de_control/ModelProces 3/Randament ==
  "q " : Inport
  um : Inport  Port=2
  Gain : Gain  Gain=8e-5
  Product : Product
  "eta " : Outport
  wires:
  um/1 -> Gain/1
  Gain/1 -> Product/2
  "q "/1 -> Product/1
  Product/1 -> "eta "/1

== system structuri_avansate_de_control/ModelProces 3/Rezervor ==
  q : Inport
  Gain : Gain  Gain=1/332.5
  Integrator : Integrator  InitialCondition=13.98
  Product : Product
  Sqrt : Sqrt
  Sum : Sum  Inputs=|+-
  c : Constant  Value=C
  h : Outport
  wires:
  Sum/1 -> Gain/1
  Sqrt/1 -> Product/1
  q/1 -> Sum/1
  Gain/1 -> Integrator/1
  Product/1 -> Sum/2
  c/1 -> Product/2
  Integrator/1 -> h/1, Sqrt/1

== system structuri_avansate_de_control/cascada/Amplificator  ==
  ua : Inport
  Constant : Constant  Value=8.1
  Gain : Gain  Gain=2.2
  Gain1 : Gain  Gain=2.2
  Gain2 : Gain  Gain=5
  Saturation : Saturate  UpperLimit=22  LowerLimit=0
  Sum : Sum  Inputs=|++
  Sum1 : Sum  Inputs=|+-
  Switch : Switch  Threshold=8.1  SaturateOnIntegerOverflow=off  InputSameDT=off
  "um " : Outport
  wires:
  Sum1/1 -> Gain2/1
  ua/1 -> Switch/2, Gain/1, Sum1/1, Gain1/1
  Gain2/1 -> Sum/2
  Gain1/1 -> Sum/1
  Sum/1 -> Switch/1
  Gain/1 -> Switch/3
  Constant/1 -> Sum1/2
  Switch/1 -> Saturation/1
  Saturation/1 -> "um "/1

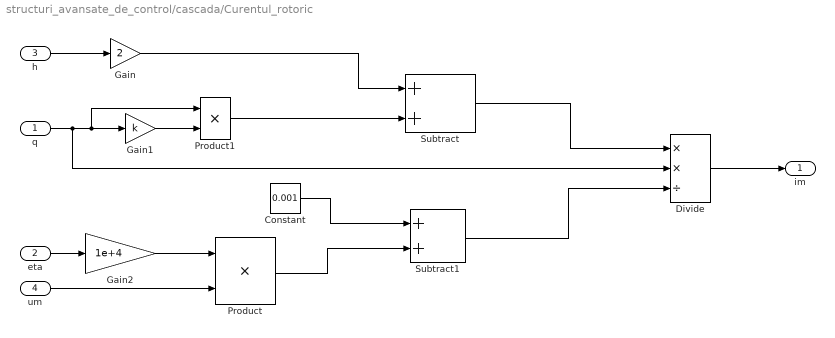
== system structuri_avansate_de_control/cascada/Curentul_rotoric ==
  q : Inport
  eta : Inport  Port=2
  h : Inport  Port=3
  um : Inport  Port=4
  Constant : Constant  Value=0.001
  Divide : Product  Inputs=**/
  Gain : Gain  Gain=2
  Gain1 : Gain  Gain=k
  Gain2 : Gain  Gain=1e+4
  Product : Product
  Product1 : Product
  Subtract : Sum
  Subtract1 : Sum
  im : Outport
  wires:
  h/1 -> Gain/1
  Gain/1 -> Subtract/1
  q/1 -> Divide/2, Product1/1, Gain1/1
  Gain1/1 -> Product1/2
  Product1/1 -> Subtract/2
  eta/1 -> Gain2/1
  Gain2/1 -> Product/1
  um/1 -> Product/2
  Constant/1 -> Subtract1/1
  Product/1 -> Subtract1/2
  Divide/1 -> im/1
  Subtract/1 -> Divide/1
  Subtract1/1 -> Divide/3

== system structuri_avansate_de_control/cascada/Filtru ==
  q : Inport
  Integrator : Integrator  InitialCondition=20.97
  Sum : Sum  Inputs=|+-
  q_f : Outport
  wires:
  Integrator/1 -> Sum/2, q_f/1
  q/1 -> Sum/1
  Sum/1 -> Integrator/1

== system structuri_avansate_de_control/cascada/Motor  ==
  um : Inport
  im : Inport  Port=2
  Add : Sum  Inputs=+-
  Rm : Gain  Gain=3
  kn : Outport
  wires:
  Rm/1 -> Add/2
  um/1 -> Add/1
  im/1 -> Rm/1
  Add/1 -> kn/1

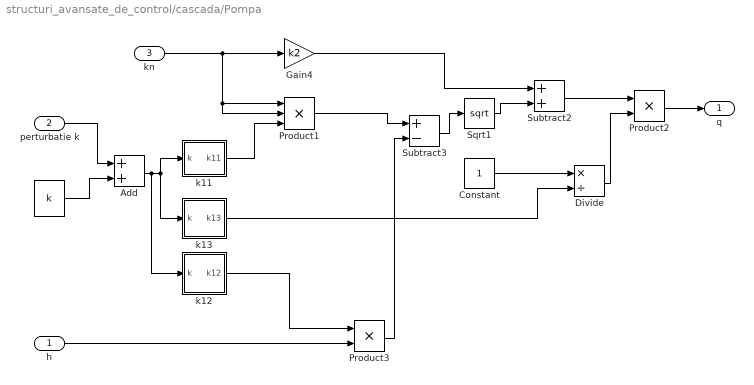
== system structuri_avansate_de_control/cascada/Pompa ==
  h : Inport
  perturbatie k : Inport  Port=2
  kn : Inport  Port=3
  " " : Constant  Value=k
  Add : Sum
  Constant : Constant
  Divide : Product  Inputs=*/
  Gain4 : Gain  Gain=k2
  Product1 : Product  Inputs=3
  Product2 : Product
  Product3 : Product
  Sqrt1 : Sqrt
  Subtract2 : Sum
  Subtract3 : Sum  Inputs=+-
  "k11 " : Subsystem
  k12 : Subsystem
  k13 : Subsystem
  q : Outport
  wires:
  Product2/1 -> q/1
  Divide/1 -> Product2/2
  Sqrt1/1 -> Subtract2/2
  k13/1(k13) -> Divide/2
  Constant/1 -> Divide/1
  "k11 "/1(k11) -> Product1/3
  Product3/1 -> Subtract3/2
  k12/1(k12) -> Product3/1
  Subtract2/1 -> Product2/1
  Add/1 -> k12/1(k), k13/1(k), "k11 "/1(k)
  perturbatie k/1 -> Add/1
  " "/1 -> Add/2
  Subtract3/1 -> Sqrt1/1
  kn/1 -> Product1/2, Product1/1, Gain4/1
  h/1 -> Product3/2
  Gain4/1 -> Subtract2/1
  Product1/1 -> Subtract3/1

== system structuri_avansate_de_control/cascada/Randament ==
  "q " : Inport
  um : Inport  Port=2
  Gain : Gain  Gain=8e-5
  Product : Product
  "eta " : Outport
  wires:
  um/1 -> Gain/1
  Gain/1 -> Product/2
  "q "/1 -> Product/1
  Product/1 -> "eta "/1

== system structuri_avansate_de_control/cascada/Rezervor ==
  q : Inport
  Gain : Gain  Gain=1/332.5
  Integrator : Integrator  InitialCondition=13.98
  Product : Product
  Sqrt : Sqrt
  Sum : Sum  Inputs=|+-
  c : Constant  Value=C
  h : Outport
  wires:
  Sum/1 -> Gain/1
  Sqrt/1 -> Product/1
  q/1 -> Sum/1
  Gain/1 -> Integrator/1
  Product/1 -> Sum/2
  c/1 -> Product/2
  Integrator/1 -> h/1, Sqrt/1

== system structuri_avansate_de_control/initial/Amplificator ==
  ua : Inport
  Constant : Constant  Value=8.1
  Gain : Gain  Gain=2.2
  Gain1 : Gain  Gain=5
  Gain2 : Gain  Gain=2.2
  Saturation : Saturate  UpperLimit=22  LowerLimit=0
  Sum : Sum  Inputs=|++
  Sum1 : Sum  Inputs=|+-
  Switch : Switch  Criteria=u2 > Threshold  Threshold=8.1  SaturateOnIntegerOverflow=off  InputSameDT=off
  um : Outport
  wires:
  Gain/1 -> Switch/3
  Sum1/1 -> Gain1/1
  ua/1 -> Gain/1, Sum1/1, Gain2/1, Switch/2
  Switch/1 -> Saturation/1
  Gain1/1 -> Sum/2
  Saturation/1 -> um/1
  Constant/1 -> Sum1/2
  Gain2/1 -> Sum/1
  Sum/1 -> Switch/1

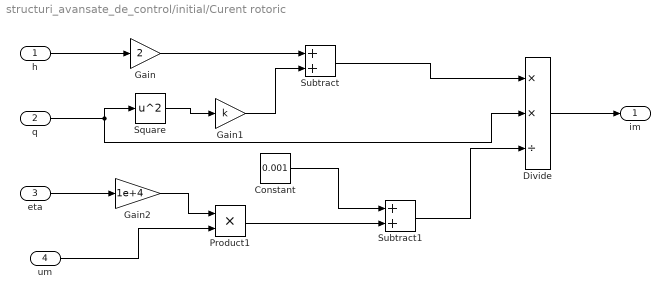
== system structuri_avansate_de_control/initial/Curent rotoric ==
  h : Inport
  q : Inport  Port=2
  eta : Inport  Port=3
  um : Inport  Port=4
  Constant : Constant  Value=0.001
  Divide : Product  Inputs=**/
  Gain : Gain  Gain=2
  Gain1 : Gain  Gain=k
  Gain2 : Gain  Gain=1e+4
  Product1 : Product
  Square : Math  Operator=square
  Subtract : Sum
  Subtract1 : Sum
  im : Outport
  wires:
  h/1 -> Gain/1
  Divide/1 -> im/1
  q/1 -> Divide/2, Square/1
  eta/1 -> Gain2/1
  um/1 -> Product1/2
  Gain2/1 -> Product1/1
  Subtract/1 -> Divide/1
  Constant/1 -> Subtract1/1
  Product1/1 -> Subtract1/2
  Subtract1/1 -> Divide/3
  Gain/1 -> Subtract/1
  Gain1/1 -> Subtract/2
  Square/1 -> Gain1/1

== system structuri_avansate_de_control/initial/Filtru ==
  q1 : Inport
  Integrator1 : Integrator  InitialCondition=q0
  Sum1 : Sum  Inputs=|+-
  q2 : Outport
  wires:
  Integrator1/1 -> q2/1, Sum1/2
  q1/1 -> Sum1/1
  Sum1/1 -> Integrator1/1

== system structuri_avansate_de_control/initial/Motor ==
  um : Inport
  im : Inport  Port=2
  Add : Sum  Inputs=+-
  Rm : Gain  Gain=3
  kn : Outport
  wires:
  Rm/1 -> Add/2
  um/1 -> Add/1
  im/1 -> Rm/1
  Add/1 -> kn/1

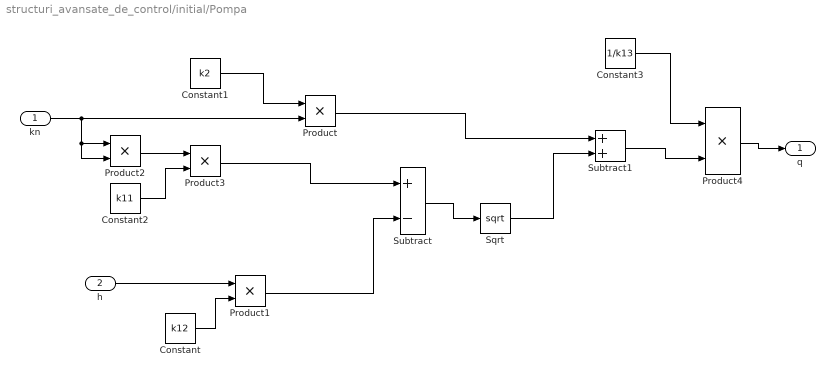
== system structuri_avansate_de_control/initial/Pompa ==
  kn : Inport
  h : Inport  Port=2
  Constant : Constant  Value=k12
  Constant1 : Constant  Value=k2
  Constant2 : Constant  Value=k11
  Constant3 : Constant  Value=1/k13
  Product{,1..4} (5 alike) : Product
  Sqrt : Sqrt
  Subtract : Sum  Inputs=+-
  Subtract1 : Sum
  q : Outport
  wires:
  Subtract/1 -> Sqrt/1
  Sqrt/1 -> Subtract1/2
  h/1 -> Product1/1
  Product1/1 -> Subtract/2
  Constant/1 -> Product1/2
  Constant1/1 -> Product/1
  kn/1 -> Product2/2, Product2/1, Product/2
  Product/1 -> Subtract1/1
  Product2/1 -> Product3/1
  Constant2/1 -> Product3/2
  Product3/1 -> Subtract/1
  Constant3/1 -> Product4/1
  Subtract1/1 -> Product4/2
  Product4/1 -> q/1

== system structuri_avansate_de_control/initial/Randament pompa ==
  q : Inport
  um : Inport  Port=2
  Gain : Gain  Gain=8e-5
  Product : Product
  eta : Outport
  wires:
  um/1 -> Gain/1
  Gain/1 -> Product/2
  q/1 -> Product/1
  Product/1 -> eta/1

== system structuri_avansate_de_control/initial/Rezervor ==
  ln1 : Inport
  Gain : Gain  Gain=1/332.5
  Gain1 : Gain  Gain=C
  Integrator1 : Integrator  InitialCondition=h0
  Sqrt : Sqrt
  Sum1 : Sum  Inputs=|+-
  h : Outport
  wires:
  Gain/1 -> Integrator1/1
  Integrator1/1 -> Sqrt/1, h/1
  Sum1/1 -> Gain/1
  ln1/1 -> Sum1/1
  Sqrt/1 -> Gain1/1
  Gain1/1 -> Sum1/2

== system structuri_avansate_de_control/perturbatie intrare + iesire/Amplificator ==
  ua : Inport
  Constant : Constant  Value=8.1
  Gain : Gain  Gain=2.2
  Gain1 : Gain  Gain=5
  Gain2 : Gain  Gain=2.2
  Saturation : Saturate  UpperLimit=22  LowerLimit=0
  Sum : Sum  Inputs=|++
  Sum1 : Sum  Inputs=|+-
  Switch : Switch  Criteria=u2 > Threshold  Threshold=8.1  SaturateOnIntegerOverflow=off  InputSameDT=off
  um : Outport
  wires:
  Gain/1 -> Switch/3
  Sum1/1 -> Gain1/1
  ua/1 -> Gain/1, Sum1/1, Gain2/1, Switch/2
  Switch/1 -> Saturation/1
  Gain1/1 -> Sum/2
  Saturation/1 -> um/1
  Constant/1 -> Sum1/2
  Gain2/1 -> Sum/1
  Sum/1 -> Switch/1

== system structuri_avansate_de_control/perturbatie intrare + iesire/Curent rotoric ==
  h : Inport
  q : Inport  Port=2
  eta : Inport  Port=3
  um : Inport  Port=4
  Constant : Constant  Value=0.001
  Divide : Product  Inputs=**/
  Gain : Gain  Gain=2
  Gain1 : Gain  Gain=k
  Gain2 : Gain  Gain=1e+4
  Product1 : Product
  Square : Math  Operator=square
  Subtract : Sum
  Subtract1 : Sum
  im : Outport
  wires:
  h/1 -> Gain/1
  Divide/1 -> im/1
  q/1 -> Divide/2, Square/1
  eta/1 -> Gain2/1
  um/1 -> Product1/2
  Gain2/1 -> Product1/1
  Subtract/1 -> Divide/1
  Constant/1 -> Subtract1/1
  Product1/1 -> Subtract1/2
  Subtract1/1 -> Divide/3
  Gain/1 -> Subtract/1
  Gain1/1 -> Subtract/2
  Square/1 -> Gain1/1

== system structuri_avansate_de_control/perturbatie intrare + iesire/Filtru ==
  q1 : Inport
  Integrator1 : Integrator  InitialCondition=20.97
  Sum1 : Sum  Inputs=|+-
  q2 : Outport
  wires:
  Integrator1/1 -> q2/1, Sum1/2
  q1/1 -> Sum1/1
  Sum1/1 -> Integrator1/1

== system structuri_avansate_de_control/perturbatie intrare + iesire/Motor ==
  um : Inport
  im : Inport  Port=2
  Add : Sum  Inputs=+-
  Rm : Gain  Gain=3
  kn : Outport
  wires:
  Rm/1 -> Add/2
  um/1 -> Add/1
  im/1 -> Rm/1
  Add/1 -> kn/1

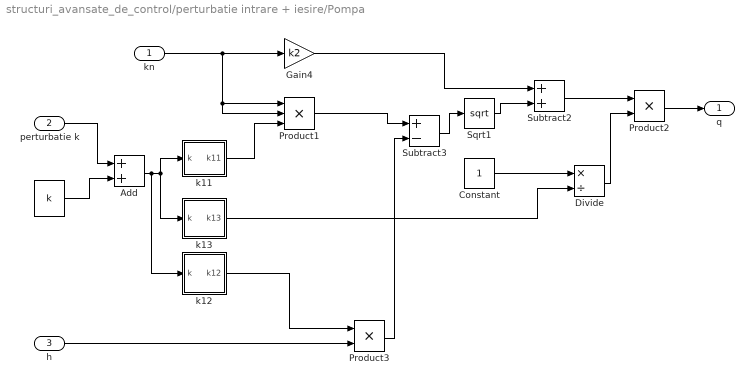
== system structuri_avansate_de_control/perturbatie intrare + iesire/Pompa ==
  kn : Inport
  perturbatie k : Inport  Port=2
  h : Inport  Port=3
  " " : Constant  Value=k
  Add : Sum
  Constant : Constant
  Divide : Product  Inputs=*/
  Gain4 : Gain  Gain=k2
  Product1 : Product  Inputs=3
  Product2 : Product
  Product3 : Product
  Sqrt1 : Sqrt
  Subtract2 : Sum
  Subtract3 : Sum  Inputs=+-
  "k11 " : Subsystem
  k12 : Subsystem
  k13 : Subsystem
  q : Outport
  wires:
  Product3/1 -> Subtract3/2
  Product1/1 -> Subtract3/1
  kn/1 -> Product1/2, Product1/1, Gain4/1
  " "/1 -> Add/2
  Constant/1 -> Divide/1
  k13/1(k13) -> Divide/2
  Add/1 -> k12/1(k), k13/1(k), "k11 "/1(k)
  Divide/1 -> Product2/2
  Subtract3/1 -> Sqrt1/1
  k12/1(k12) -> Product3/1
  Sqrt1/1 -> Subtract2/2
  "k11 "/1(k11) -> Product1/3
  h/1 -> Product3/2
  Subtract2/1 -> Product2/1
  Gain4/1 -> Subtract2/1
  perturbatie k/1 -> Add/1
  Product2/1 -> q/1

== system structuri_avansate_de_control/perturbatie intrare + iesire/Randament pompa ==
  q : Inport
  um : Inport  Port=2
  Gain : Gain  Gain=8e-5
  Product : Product
  eta : Outport
  wires:
  um/1 -> Gain/1
  Gain/1 -> Product/2
  q/1 -> Product/1
  Product/1 -> eta/1

== system structuri_avansate_de_control/perturbatie intrare + iesire/Rezervor ==
  q : Inport
  Add : Sum
  Constant : Constant  Value=C
  Gain : Gain  Gain=1/332.5
  Integrator1 : Integrator  InitialCondition=13.98
  Product : Product
  Product1 : Product
  Scope : Scope
  Sqrt : Sqrt
  Step : Step  Time=400  SampleTime=0
  Sum1 : Sum  Inputs=|+-
  h : Outport
  perturbatie : Outport  Port=2
  wires:
  Gain/1 -> Integrator1/1
  Integrator1/1 -> Sqrt/1, h/1
  Sum1/1 -> Gain/1
  q/1 -> Sum1/1
  Sqrt/1 -> Product1/1, Product/1
  Product/1 -> Sum1/2, Scope/1
  Product1/1 -> perturbatie/1
  Constant/1 -> Add/2
  Step/1 -> Product1/2, Add/1
  Add/1 -> Product/2

== system structuri_avansate_de_control/ModelProces 2/Pompa/k11  ==
  k : Inport
  Add : Sum
  Constant : Constant  Value=4
  Product : Product
  Product1 : Product  Inputs=3
  Subtract : Sum  Inputs=+-
  k1 : Constant  Value=k1
  k2 : Constant  Value=k2
  k3 : Constant  Value=k3
  k11 : Outport
  wires:
  k2/1 -> Product/2, Product/1
  k/1 -> Subtract/1
  k3/1 -> Subtract/2
  Subtract/1 -> Product1/1
  k1/1 -> Product1/2
  Constant/1 -> Product1/3
  Product1/1 -> Add/1
  Product/1 -> Add/2
  Add/1 -> k11/1

== system structuri_avansate_de_control/ModelProces 2/Pompa/k12 ==
  k : Inport
  Product1 : Product
  Subtract : Sum  Inputs=+-
  "constant " : Constant  Value=8
  k3 : Constant  Value=k3
  k12 : Outport
  wires:
  k/1 -> Subtract/1
  k3/1 -> Subtract/2
  Subtract/1 -> Product1/1
  "constant "/1 -> Product1/2
  Product1/1 -> k12/1

== system structuri_avansate_de_control/ModelProces 2/Pompa/k13 ==
  k : Inport
  Product1 : Product
  Subtract : Sum  Inputs=+-
  "constant " : Constant  Value=2
  k3 : Constant  Value=k3
  k13 : Outport
  wires:
  k/1 -> Subtract/1
  k3/1 -> Subtract/2
  Subtract/1 -> Product1/1
  "constant "/1 -> Product1/2
  Product1/1 -> k13/1

== system structuri_avansate_de_control/ModelProces 3/Pompa/k11  ==
  k : Inport
  Add : Sum
  Constant : Constant  Value=4
  Product : Product
  Product1 : Product  Inputs=3
  Subtract : Sum  Inputs=+-
  k1 : Constant  Value=k1
  k2 : Constant  Value=k2
  k3 : Constant  Value=k3
  k11 : Outport
  wires:
  k2/1 -> Product/2, Product/1
  k/1 -> Subtract/1
  k3/1 -> Subtract/2
  Subtract/1 -> Product1/1
  k1/1 -> Product1/2
  Constant/1 -> Product1/3
  Product1/1 -> Add/1
  Product/1 -> Add/2
  Add/1 -> k11/1
